simulink model "BLAC_MotorCtrl_Math"  (R2023b)
settings: Solver=FixedStepDiscrete  StartTime=0.0  StopTime=0.1  FixedStep=MC_Sim_BaseStep  RelTol=1e-3  EnableMultiTasking=on
values from neighbouring files (symbols this model uses):
  MC_Hardware_Chip_ADCResultBit = 0.0    [MotorControlDataDictionary_Math.sldd]
  MC_Hardware_Chip_ADCVoltageMax = 1.0    [MotorControlDataDictionary_Math.sldd]
  MC_Hardware_Chip_ADCVoltageRefence = 0.0    [MotorControlDataDictionary_Math.sldd]
  MC_Hardware_Chip_CSAGain = 1.0    [MotorControlDataDictionary_Math.sldd]
  MC_Hardware_Sample_Resistor = 0.001    [MotorControlDataDictionary_Math.sldd]
  MC_MotorModel_Machine_Damp = 0.0    [MotorControlDataDictionary_Math.sldd]
  MC_MotorModel_Machine_Ineria = 0.0    [MotorControlDataDictionary_Math.sldd]
  MC_MotorModel_Machine_Tfric = 0.0    [MotorControlDataDictionary_Math.sldd]
  MC_MotorModel_Rotor_Pn = 4.0    [MotorControlDataDictionary_Math.sldd]
  MC_MotorModel_Stator_Ld = 0.0    [MotorControlDataDictionary_Math.sldd]
  MC_MotorModel_Stator_Lq = 0.0    [MotorControlDataDictionary_Math.sldd]
  MC_MotorModel_Stator_Rs = 1.0    [MotorControlDataDictionary_Math.sldd]
  MC_Sim_BaseStep = 2.5E-8    [MotorControlDataDictionary_Math.sldd]
  MC_Sim_HFTStep = 6.6675E-5    [MotorControlDataDictionary_Math.sldd]
undefined symbols (not defined in the file or in its folder): MC_MOS_DeadTime, MC_Motor_Phi, MC_Motor_Rotor_Pn, MC_Motor_Stator_Ld, MC_Motor_Stator_Lq, MC_Motor_Stator_Rs, MC_Param_CurrentPI_Ki, MC_Param_CurrentPI_Kp, MC_Param_CurrentPI_UdInteMax, MC_Param_CurrentPI_UdInteMin, MC_Param_CurrentPI_UdMax, MC_Param_CurrentPI_UdMin, MC_Param_CurrentPI_UqInteMax, MC_Param_CurrentPI_UqInteMin, MC_Param_CurrentPI_UqMax, MC_Param_CurrentPI_UqMin, MC_Param_Flux_Gamma, MC_Param_Flux_Lalpha, MC_Param_Flux_Lbeta, MC_Param_Flux_Ralpha, MC_Param_Flux_Rbeta, MC_Param_Luen_BEMFalpha, MC_Param_Luen_BEMFbeta, MC_Param_Luen_BEMFErr, MC_Param_Luen_Currentalpha, MC_Param_Luen_Currentbeta, MC_Param_Luen_CurrentErr, MC_Param_Luen_PLL_Ki, MC_Param_Luen_PLL_Kp, MC_Param_Luen_Voltagealpha, MC_Param_Luen_Voltagebeta, MC_Param_PhasetoReal, MC_Param_SMO_CoffA, MC_Param_SMO_CoffB, MC_Param_SpeedtoTheta, MC_Param_SVPWM_DutyMax, MC_Param_SVPWM_DutyMin, MC_Param_SVPWM_SampleOffset1, MC_Param_SVPWM_SampleOffset2, MC_Param_SVPWM_SampleValid
libraries: simulink x29, spsSeriesRLCBranchLib x6, spsVoltageMeasurementLib x6, spsIGBTLib x6, spsDiodeLib x4, spsACVoltageSourceLib x1, spsGroundLib x1, spsPermanentMagnetSynchronousMachineLib x1, spsThreePhaseVIMeasurementLib x1, spspowerguiLib x1
(part 2 of 3)

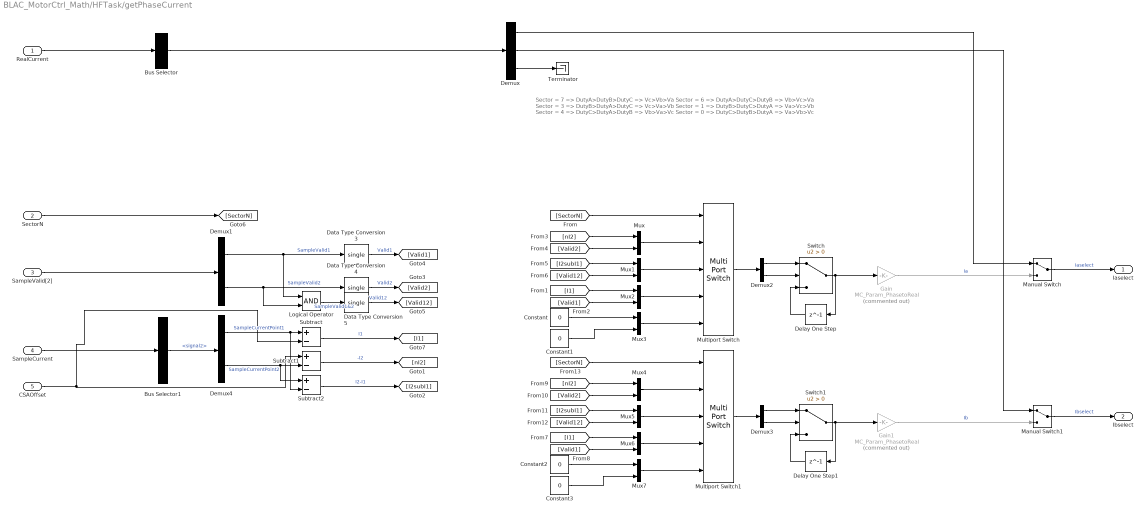
== system BLAC_MotorCtrl_Math/HFTask/getPhaseCurrent ==
  note: Sector = 7 => DutyA>DutyB>DutyC => Vc>Vb>Va
      | Sector = 6 => DutyA>DutyC>DutyB => Vb>Vc>Va
      | Sector = 3 => DutyB>DutyA>DutyC => Vc>Va>Vb
      | Sector = 1 => DutyB>DutyC>DutyA => Va>Vc>Vb
      | Sector = 4 => DutyC>DutyA>DutyB => Vb>Va>Vc
      | Sector = 0 => DutyC>DutyB>DutyA => Va>Vb>Vc
  RealCurrent : Inport
  SectorN : Inport  Port=2
  SampleValid[2] : Inport  Port=3
  SampleCurrent : Inport  Port=4
  CSAOffset : Inport  Port=5
  Bus Selector : BusSelector  OutputSignals=PhaseI  OutputAsBus=on
  Bus Selector1 : BusSelector  OutputSignals=signal2
  Constant{,1..3} (4 alike) : Constant  Value=0  OutDataTypeStr=single
  Data Type Conversion3 : DataTypeConversion  OutDataTypeStr=single  RndMeth=Simplest  SaturateOnIntegerOverflow=off
  Data Type Conversion4 : DataTypeConversion  OutDataTypeStr=single  RndMeth=Simplest  SaturateOnIntegerOverflow=off
  Data Type Conversion5 : DataTypeConversion  OutDataTypeStr=single  RndMeth=Simplest  SaturateOnIntegerOverflow=off
  Delay One Step : Delay  DelayLength=1
  Delay One Step1 : Delay  DelayLength=1
  Demux : Demux  Outputs=3
  Demux{1..4} (4 alike) : Demux  Outputs=2
  Gain : Gain  Commented=on  Gain=MC_Param_PhasetoReal
  Gain1 : Gain  Commented=on  Gain=MC_Param_PhasetoReal
  Logical Operator : Logic  AllPortsSameDT=off  OutDataTypeStr=boolean
  Manual Switch : ManualSwitch
  Manual Switch1 : ManualSwitch
  Multiport Switch : MultiPortSwitch  DataPortOrder=Specify indices  DataPortIndices={[7,6],[3,4],[0,1]}  DataPortForDefault=Additional data port  SaturateOnIntegerOverflow=off  InputSameDT=off
  Multiport Switch1 : MultiPortSwitch  DataPortOrder=Specify indices  DataPortIndices={[3,1],[7,0],[6,4]}  DataPortForDefault=Additional data port  SaturateOnIntegerOverflow=off  InputSameDT=off
  Mux{,1..7} (8 alike) : Mux  Inputs=2
  Subtract : Sum  Inputs=+-
  Subtract1 : Sum  Inputs=+-
  Subtract2 : Sum  Inputs=+-
  Switch : Switch  Criteria=u2 > Threshold  SaturateOnIntegerOverflow=off  InputSameDT=off
  Switch1 : Switch  Criteria=u2 > Threshold  SaturateOnIntegerOverflow=off  InputSameDT=off
  Terminator : Terminator
  Iaselect : Outport
  Ibselect : Outport  Port=2
  wires:
  RealCurrent/1 -> Bus Selector/1
  Bus Selector/1 -> Demux/1
  Manual Switch/1 -> Iaselect/1  "Iaselect"
  Demux/3 -> Terminator/1
  Manual Switch1/1 -> Ibselect/1  "Ibselect"
  Multiport Switch1/1 -> Demux3/1
  Demux3/2 -> Switch1/2
  Demux3/1 -> Switch1/1
  Switch1/1 -> Delay One Step1/1, Gain1/1
  Delay One Step1/1 -> Switch1/3
  Gain1/1 -> Manual Switch1/2  "Ib"
  Gain/1 -> Manual Switch/2  "Ia"
  Delay One Step/1 -> Switch/3
  Switch/1 -> Gain/1, Delay One Step/1
  Demux2/1 -> Switch/1
  Demux2/2 -> Switch/2
  Multiport Switch/1 -> Demux2/1
  [SectorN] -> Multiport Switch1/1
  Mux4/1 -> Multiport Switch1/2
  Mux5/1 -> Multiport Switch1/3
  Mux6/1 -> Multiport Switch1/4
  [I1] -> Mux6/1
  [Valid1] -> Mux6/2
  [nI2] -> Mux4/1
  [Valid2] -> Mux4/2
  [Valid12] -> Mux5/2
  [I2subI1] -> Mux5/1
  Mux7/1 -> Multiport Switch1/5
  Constant2/1 -> Mux7/1
  Constant3/1 -> Mux7/2
  Subtract/1 -> [I1]  "I1"
  Subtract1/1 -> [nI2]  "-I2"
  Data Type Conversion5/1 -> [Valid12]  "Valid12"
  Data Type Conversion4/1 -> [Valid2]  "Valid2"
  Data Type Conversion3/1 -> [Valid1]  "Valid1"
  Subtract2/1 -> [I2subI1]  "I2-I1"
  Constant1/1 -> Mux3/2
  Constant/1 -> Mux3/1
  Mux3/1 -> Multiport Switch/5
  [I2subI1] -> Mux1/1
  [Valid12] -> Mux1/2
  [Valid2] -> Mux/2
  [nI2] -> Mux/1
  [Valid1] -> Mux2/2
  [I1] -> Mux2/1
  [SectorN] -> Multiport Switch/1
  SectorN/1 -> [SectorN]
  Mux2/1 -> Multiport Switch/4
  Mux1/1 -> Multiport Switch/3
  Mux/1 -> Multiport Switch/2
  Logical Operator/1 -> Data Type Conversion5/1  "SampleValid1&2"
  Demux1/2 -> Data Type Conversion4/1, Logical Operator/2  "SampleValid2"
  Demux1/1 -> Data Type Conversion3/1, Logical Operator/1  "SampleValid1"
  SampleValid[2]/1 -> Demux1/1
  Demux4/2 -> Subtract2/1, Subtract1/2  "SampleCurrentPoint2"
  CSAOffset/1 -> Subtract1/1, Subtract/2
  Demux4/1 -> Subtract2/2, Subtract/1  "SampleCurrentPoint1"
  Bus Selector1/1 -> Demux4/1  "<signal2>"
  SampleCurrent/1 -> Bus Selector1/1
  Demux/1 -> Manual Switch/1
  Demux/2 -> Manual Switch1/1

== system BLAC_MotorCtrl_Math/HFTask/getSinCos ==
  Theta : Inport
  Sin : Trigonometry
  Sin1 : Trigonometry  Operator=cos
  SinTheta : Outport
  CosTheta : Outport  Port=2
  wires:
  Theta/1 -> Sin1/1, Sin/1
  Sin/1 -> SinTheta/1
  Sin1/1 -> CosTheta/1

== system BLAC_MotorCtrl_Math/HFTask/invParkTransform ==
  Ud : Inport
  Uq : Inport  Port=2
  SinTheta : Inport  Port=3
  CosTheta : Inport  Port=4
  Add : Sum
  Product{,1..3} (4 alike) : Product
  Subtract : Sum  Inputs=+-
  Ualpha : Outport
  Ubeta : Outport  Port=2
  wires:
  Uq/1 -> Product3/1, Product1/1
  Subtract/1 -> Ualpha/1  "Ualpha"
  CosTheta/1 -> Product/2, Product3/2
  SinTheta/1 -> Product2/2, Product1/2
  Product/1 -> Subtract/1
  Product1/1 -> Subtract/2
  Ud/1 -> Product/1, Product2/1
  Product2/1 -> Add/1
  Product3/1 -> Add/2
  Add/1 -> Ubeta/1  "Ubeta"

== system BLAC_MotorCtrl_Math/HFTask/karmalObservor ==
  In1 : Inport
  Out1 : Outport
  wires:
  In1/1 -> Out1/1

== system BLAC_MotorCtrl_Math/HFTask/scvmobservor ==
  Vd : Inport
  Vq : Inport  Port=2
  Id : Inport  Port=3
  Iq : Inport  Port=4
  getW : Subsystem
  wires:
  Vd/1 -> getW/1(Vd)
  Vq/1 -> getW/2(Vq)
  Id/1 -> getW/3(Id)
  Iq/1 -> getW/4(Iq)

== system BLAC_MotorCtrl_Math/HFTask/smo ==
  Valpha : Inport
  Vbeta : Inport  Port=2
  Ialpha : Inport  Port=3
  Ibeta : Inport  Port=4
  getE : Subsystem
  getSpeedandTheta : Subsystem
  Speed : Outport
  Theta : Outport  Port=2
  wires:
  Valpha/1 -> getE/1(Valpha)
  Vbeta/1 -> getE/2(Vbeta)
  Ialpha/1 -> getE/3(Ialpha)
  Ibeta/1 -> getE/4(Ibeta)
  getE/1(Ealpha) -> getSpeedandTheta/1(Ealpha)
  getE/2(Ebeta) -> getSpeedandTheta/2(Ebeta)
  getSpeedandTheta/1(Speed) -> Speed/1
  getSpeedandTheta/2(Theta) -> Theta/1

== system BLAC_MotorCtrl_Math/HFTask/svpwm ==
  Valpha : Inport
  Vbeta : Inport  Port=2
  Vdc : Inport  Port=3
  Ia : Inport  Port=4
  Ib : Inport  Port=5
  PhaseShortEnableFlag : Inport  Port=6
  Terminator : Terminator
  getVoltageExchange : Subsystem
  setDTCompelte : Subsystem
  setPhaseandSample_ORS_Double : Subsystem
  setPhaseandSample_ORS_Double1 : Subsystem  Commented=on
  DutySVPWM : Outport
  SamplePoint : Outport  Port=2
  SampleValid : Outport  Port=3
  SectorN : Outport  Port=4
  wires:
  Valpha/1 -> getVoltageExchange/1(Valpha)
  Vbeta/1 -> getVoltageExchange/2(Vbeta)
  Vdc/1 -> getVoltageExchange/3(Vdc)
  getVoltageExchange/1(Va) -> setDTCompelte/1(Va)
  getVoltageExchange/2(Vb) -> setDTCompelte/2(Vb)
  getVoltageExchange/3(Vc) -> setDTCompelte/3(Vc)
  getVoltageExchange/4(Vmed) -> setDTCompelte/4(Vmed)
  Ia/1 -> setDTCompelte/5(Ia)
  Ib/1 -> setDTCompelte/6(ib)
  setDTCompelte/1(SectorN) -> SectorN/1, setPhaseandSample_ORS_Double/1(SectorN)
  setDTCompelte/2(DutyLMS) -> setPhaseandSample_ORS_Double/2(DutyLMS)
  setPhaseandSample_ORS_Double/1(DutySVPWM) -> DutySVPWM/1
  setPhaseandSample_ORS_Double/2(SamplePoint) -> SamplePoint/1
  setPhaseandSample_ORS_Double/3(SampleValid) -> SampleValid/1
  PhaseShortEnableFlag/1 -> Terminator/1

== system BLAC_MotorCtrl_Math/HFTask/voltageLimit ==
  UdRef : Inport
  UqRef : Inport  Port=2
  Umax : Inport  Port=3
  Add : Sum
  Compare To Constant : simulink/Logic and Bit Operations/Compare To Constant  relop=<=  const=0  OutDataTypeStr=boolean
  Compare To Constant1 : simulink/Logic and Bit Operations/Compare To Constant  relop=>=  const=0  OutDataTypeStr=boolean
  Constant : Constant  Value=0  OutDataTypeStr=single
  Gain : Gain  Gain=-1
  Gain1 : Gain  Gain=-1
  Product : Product
  Saturation Dynamic : simulink/Discontinuities/Saturation Dynamic  OutMin=[]  OutMax=[]  OutDataTypeStr=Inherit: Same as second input  OutDataType=fixdt(1, 16)  OutScaling=2^-10  DoSatur=off
  Sqrt : Sqrt
  Subtract : Sum  Inputs=+-
  Switch : Switch  Criteria=u2 > Threshold  SaturateOnIntegerOverflow=off  InputSameDT=off
  Switch1 : Switch  Criteria=u2 > Threshold  SaturateOnIntegerOverflow=off  InputSameDT=off
  Switch2 : Switch  Criteria=u2 > Threshold  SaturateOnIntegerOverflow=off  InputSameDT=off
  Ud : Outport
  Uq : Outport  Port=2
  wires:
  Add/1 -> Product/1
  Subtract/1 -> Product/2
  Product/1 -> Compare To Constant/1, Sqrt/1
  Compare To Constant/1 -> [UdOverFlow]
  Sqrt/1 -> Gain/1, Saturation Dynamic/1
  Gain/1 -> Saturation Dynamic/3
  UdRef/1 -> [UdRef]
  UqRef/1 -> [UqRef]
  Umax/1 -> [Umax]
  [Umax] -> Subtract/1, Add/1
  [UdRef] -> Add/2, Subtract/2
  [UqRef] -> Saturation Dynamic/2
  Saturation Dynamic/1 -> Switch/3
  [UdOverFlow] -> Switch/2
  Constant/1 -> Switch/1
  Switch/1 -> Uq/1  "UqLimit"
  Switch1/1 -> Ud/1  "UdLimit"
  Switch2/1 -> Switch1/1
  [UdRef] -> Compare To Constant1/1
  Compare To Constant1/1 -> Switch2/2
  [Umax] -> Gain1/1, Switch2/1
  Gain1/1 -> Switch2/3
  [UdOverFlow] -> Switch1/2
  [UdRef] -> Switch1/3

== system BLAC_MotorCtrl_Math/Hardware_Sim/ACtoDC_Sim ==
  Diode{1..4} (4 alike) : spsDiodeLib/Diode  Ron=MC_Hardware_Diode_Rds  Lon=MC_Hardware_Diode_Lon  Vf=MC_Hardware_Diode_Vf  IC=0  UseSnubber=0  Rs=MC_Hardware_Diode_SR  Cs=MC_Hardware_Diode_SC  Measurements=off
  U : PMIOPort  Side=Left
  L : PMIOPort  Port=2  Side=Left
  VH : PMIOPort  Port=3  Side=Right
  VL : PMIOPort  Port=4  Side=Right
  connections:
  L/RConn1 -- Diode3/RConn1 -- Diode2/LConn1
  VL/RConn1 -- Diode4/LConn1 -- Diode3/LConn1
  Diode1/RConn1 -- Diode2/RConn1 -- VH/RConn1
  Diode1/LConn1 -- Diode4/RConn1 -- U/RConn1

== system BLAC_MotorCtrl_Math/Hardware_Sim/CurrentSample_Sim ==
  Current_Sample_Trigger : Inport
  ADCSample_Sim : Subsystem  Commented=on
  PhaseCurrentSmaple : Subsystem  Variant=on  VariantControl=PhaseCurrentSmaple
  Series RLC Branch{,1..3} (4 alike) : spsSeriesRLCBranchLib/Series RLC Branch  LConnTagsString=__new0  RConnTagsString=__new0  BranchType=R  Resistance=MC_Hardware_Sample_Resistor  Inductance=1e-3  SetiL0=off  InitialCurrent=0  Capacitance=1e-6  Setx0=off  InitialVoltage=0  Measurements=None
  Voltage Measurement{,1..3} (4 alike) : spsVoltageMeasurementLib/Voltage Measurement  PhasorSimulation=off  OutputType=Complex  PSBequivalent=0
  AL : PMIOPort  Side=Left
  BL : PMIOPort  Port=2  Side=Left
  CL : PMIOPort  Port=3  Side=Left
  VL : PMIOPort  Port=4  Side=Left
  Current_Sample : Outport
  wires:
  Voltage Measurement1/1 -> PhaseCurrentSmaple/4(SRV_A)
  Voltage Measurement2/1 -> PhaseCurrentSmaple/3(SRV_B)
  Voltage Measurement3/1 -> PhaseCurrentSmaple/2(SRV_C)
  Voltage Measurement/1 -> PhaseCurrentSmaple/5(ShuntV)
  Current_Sample_Trigger/1 -> PhaseCurrentSmaple/1(SampleTrigger)
  PhaseCurrentSmaple/1(CurrentSampleResult) -> Current_Sample/1
  connections:
  Series RLC Branch1/RConn1 -- Voltage Measurement1/LConn2 -- Voltage Measurement3/LConn2 -- Series RLC Branch3/RConn1 -- Voltage Measurement2/LConn2 -- Series RLC Branch2/RConn1 -- Voltage Measurement/LConn1 -- Series RLC Branch/LConn1
  Series RLC Branch2/LConn1 -- Voltage Measurement2/LConn1 -- BL/RConn1
  Series RLC Branch1/LConn1 -- Voltage Measurement1/LConn1 -- AL/RConn1
  VL/RConn1 -- Voltage Measurement/LConn2 -- Series RLC Branch/RConn1
  Series RLC Branch3/LConn1 -- Voltage Measurement3/LConn1 -- CL/RConn1

== system BLAC_MotorCtrl_Math/Hardware_Sim/DrivePWM_Sim ==
  ClockCounter : Inport
  DrivePWM : Inport  Port=2
  Data Type Conversion{,1..5} (6 alike) : DataTypeConversion  OutDataTypeStr=double  RndMeth=Simplest  SaturateOnIntegerOverflow=off
  Demux : Demux  Outputs=6
  Relational Operator : RelationalOperator  Operator=>  OutDataTypeStr=boolean  RndMeth=Simplest  InputSameDT=off
  Relational Operator1 : RelationalOperator  Operator=>  OutDataTypeStr=boolean  RndMeth=Simplest  InputSameDT=off
  Relational Operator2 : RelationalOperator  Operator=>  OutDataTypeStr=boolean  RndMeth=Simplest  InputSameDT=off
  Relational Operator3 : RelationalOperator  Operator=<  OutDataTypeStr=boolean  RndMeth=Simplest  InputSameDT=off
  Relational Operator4 : RelationalOperator  Operator=<  OutDataTypeStr=boolean  RndMeth=Simplest  InputSameDT=off
  Relational Operator5 : RelationalOperator  Operator=<  OutDataTypeStr=boolean  RndMeth=Simplest  InputSameDT=off
  Drive_A_H : Outport
  Drive_B_H : Outport  Port=2
  Drive_C_H : Outport  Port=3
  Drive_A_L : Outport  Port=4
  Drive_B_L : Outport  Port=5
  Drive_C_L : Outport  Port=6
  wires:
  Relational Operator1/1 -> Data Type Conversion1/1
  Demux/2 -> Relational Operator1/2
  Demux/5 -> Relational Operator4/2
  Demux/1 -> Relational Operator/2
  DrivePWM/1 -> Demux/1
  Relational Operator2/1 -> Data Type Conversion3/1
  ClockCounter/1 -> Relational Operator5/1, Relational Operator4/1, Relational Operator3/1, Relational Operator2/1, Relational Operator1/1, Relational Operator/1
  Demux/6 -> Relational Operator5/2
  Relational Operator/1 -> Data Type Conversion/1
  Demux/4 -> Relational Operator3/2
  Relational Operator3/1 -> Data Type Conversion2/1
  Data Type Conversion5/1 -> Drive_C_L/1
  Relational Operator5/1 -> Data Type Conversion5/1
  Demux/3 -> Relational Operator2/2
  Relational Operator4/1 -> Data Type Conversion4/1
  Data Type Conversion3/1 -> Drive_C_H/1
  Data Type Conversion4/1 -> Drive_B_L/1
  Data Type Conversion2/1 -> Drive_A_L/1
  Data Type Conversion1/1 -> Drive_B_H/1
  Data Type Conversion/1 -> Drive_A_H/1

== system BLAC_MotorCtrl_Math/Hardware_Sim/IGBT_Drive_Sim ==
  Drive_A_H : Inport
  Drive_B_H : Inport  Port=2
  Drive_C_H : Inport  Port=3
  Drive_A_L : Inport  Port=4
  Drive_B_L : Inport  Port=5
  Drive_C_L : Inport  Port=6
  IGBT{,1..5} (6 alike) : spsIGBTLib/IGBT  Ron=MC_Hardware_IGBT_Rds  Lon=MC_Hardware_IGBT_Lon  Vf=MC_Hardware_IGBT_Vf  Tf=1e-6  Tt=2e-6  IC=0  Rs=MC_Hardware_IGBT_SR  Cs=MC_Hardware_IGBT_SC  Measurements=on
  Mux : Mux  Inputs=3
  Mux1 : Mux  Inputs=3
  VH : PMIOPort  Side=Left
  A : PMIOPort  Port=2  Side=Right
  B : PMIOPort  Port=3  Side=Right
  C : PMIOPort  Port=4  Side=Right
  AL : PMIOPort  Port=5  Side=Right
  BL : PMIOPort  Port=6  Side=Right
  CL : PMIOPort  Port=7  Side=Right
  IGBT_M_H : Outport
  IGBT_M_L : Outport  Port=2
  wires:
  IGBT4/1 -> Mux/2
  Drive_C_H/1 -> IGBT2/1
  Drive_B_H/1 -> IGBT1/1
  IGBT5/1 -> Mux/1
  Drive_B_L/1 -> IGBT4/1
  Drive_A_H/1 -> IGBT/1
  Drive_C_L/1 -> IGBT5/1
  IGBT3/1 -> Mux/3
  Drive_A_L/1 -> IGBT3/1
  IGBT2/1 -> Mux1/3
  IGBT1/1 -> Mux1/2
  IGBT/1 -> Mux1/1
  Mux1/1 -> IGBT_M_H/1
  Mux/1 -> IGBT_M_L/1
  connections:
  IGBT/RConn1 -- IGBT3/LConn1 -- A/RConn1
  IGBT3/RConn1 -- AL/RConn1
  IGBT2/LConn1 -- IGBT1/LConn1 -- VH/RConn1 -- IGBT/LConn1
  C/RConn1 -- IGBT5/LConn1 -- IGBT2/RConn1
  B/RConn1 -- IGBT4/LConn1 -- IGBT1/RConn1
  IGBT5/RConn1 -- CL/RConn1
  IGBT4/RConn1 -- BL/RConn1

== system BLAC_MotorCtrl_Math/Hardware_Sim/SampleTrigger_Sim ==
  ClockCounter : Inport
  SamplePoint : Inport  Port=2
  Data Type Conversion{,1..4} (5 alike) : DataTypeConversion  OutDataTypeStr=double  RndMeth=Simplest  SaturateOnIntegerOverflow=off
  Demux : Demux  Outputs=5
  Mux : Mux  Inputs=3
  Relational Operator{,1..4} (5 alike) : RelationalOperator  Operator=>  OutDataTypeStr=boolean  RndMeth=Simplest  InputSameDT=off
  Current_Sample_Trigger : Outport
  Vbus_Sample_Trigger : Outport  Port=2
  Temp_Sample_Trigger : Outport  Port=3
  wires:
  SamplePoint/1 -> Demux/1
  Relational Operator/1 -> Data Type Conversion/1
  Demux/1 -> Relational Operator/2
  Demux/2 -> Relational Operator1/2
  Relational Operator1/1 -> Data Type Conversion1/1
  Relational Operator2/1 -> Data Type Conversion2/1
  Demux/4 -> Relational Operator2/2
  Demux/5 -> Relational Operator3/2
  Relational Operator3/1 -> Data Type Conversion3/1
  ClockCounter/1 -> Relational Operator4/1, Relational Operator3/1, Relational Operator2/1, Relational Operator1/1, Relational Operator/1
  Data Type Conversion/1 -> Mux/1
  Data Type Conversion1/1 -> Mux/2
  Mux/1 -> Current_Sample_Trigger/1
  Data Type Conversion2/1 -> Vbus_Sample_Trigger/1
  Data Type Conversion3/1 -> Temp_Sample_Trigger/1
  Demux/3 -> Relational Operator4/2
  Relational Operator4/1 -> Data Type Conversion4/1
  Data Type Conversion4/1 -> Mux/3

== system BLAC_MotorCtrl_Math/Hardware_Sim/VbusSample_Sim ==
  Vbus_Sample_Trigger : Inport
  ADCSample_Sim : Subsystem
  ADCSample_Sim1 : Subsystem
  Add1 : Sum
  Add2 : Sum
  Band-Limited White Noise : simulink/Sources/Band-Limited White Noise  Cov=MC_Sim_NoisePower_VACbus  Ts=MC_Sim_BaseStep  seed=[23222]
  Band-Limited White Noise1 : simulink/Sources/Band-Limited White Noise  Cov=MC_Sim_NoisePower_VDCbus  Ts=MC_Sim_BaseStep  seed=[23241]
  Series RLC Branch : spsSeriesRLCBranchLib/Series RLC Branch  LConnTagsString=__new0  RConnTagsString=__new0  BranchType=R  Resistance=1e3  Inductance=1e-3  SetiL0=off  InitialCurrent=0  Capacitance=1e-6  Setx0=off  InitialVoltage=0  Measurements=None
  Series RLC Branch1 : spsSeriesRLCBranchLib/Series RLC Branch  LConnTagsString=__new0  RConnTagsString=__new0  BranchType=R  Resistance=1e3  Inductance=1e-3  SetiL0=off  InitialCurrent=0  Capacitance=1e-6  Setx0=off  InitialVoltage=0  Measurements=None
  Voltage Measurement : spsVoltageMeasurementLib/Voltage Measurement  PhasorSimulation=off  OutputType=Complex  PSBequivalent=0
  Voltage Measurement1 : spsVoltageMeasurementLib/Voltage Measurement  PhasorSimulation=off  OutputType=Complex  PSBequivalent=0
  DCH : PMIOPort  Side=Left
  DCL : PMIOPort  Port=2  Side=Left
  ACH : PMIOPort  Port=3  Side=Left
  ACL : PMIOPort  Port=4  Side=Left
  Vbus_Sample_AC : Outport
  Vbus_Sample_DC : Outport  Port=2
  wires:
  ADCSample_Sim/1(Sample_Out) -> Vbus_Sample_AC/1
  ADCSample_Sim1/1(Sample_Out) -> Vbus_Sample_DC/1
  Vbus_Sample_Trigger/1 -> ADCSample_Sim1/Trigger, ADCSample_Sim/Trigger
  Band-Limited White Noise/1 -> Add1/2
  Add1/1 -> ADCSample_Sim/1(Sample_In)
  Voltage Measurement/1 -> Add1/1
  Band-Limited White Noise1/1 -> Add2/2
  Voltage Measurement1/1 -> Add2/1
  Add2/1 -> ADCSample_Sim1/1(Sample_In)
  connections:
  ACH/RConn1 -- Voltage Measurement/LConn1 -- Series RLC Branch/LConn1
  ACL/RConn1 -- Voltage Measurement/LConn2 -- Series RLC Branch/RConn1
  DCL/RConn1 -- Series RLC Branch1/RConn1 -- Voltage Measurement1/LConn2
  DCH/RConn1 -- Series RLC Branch1/LConn1 -- Voltage Measurement1/LConn1

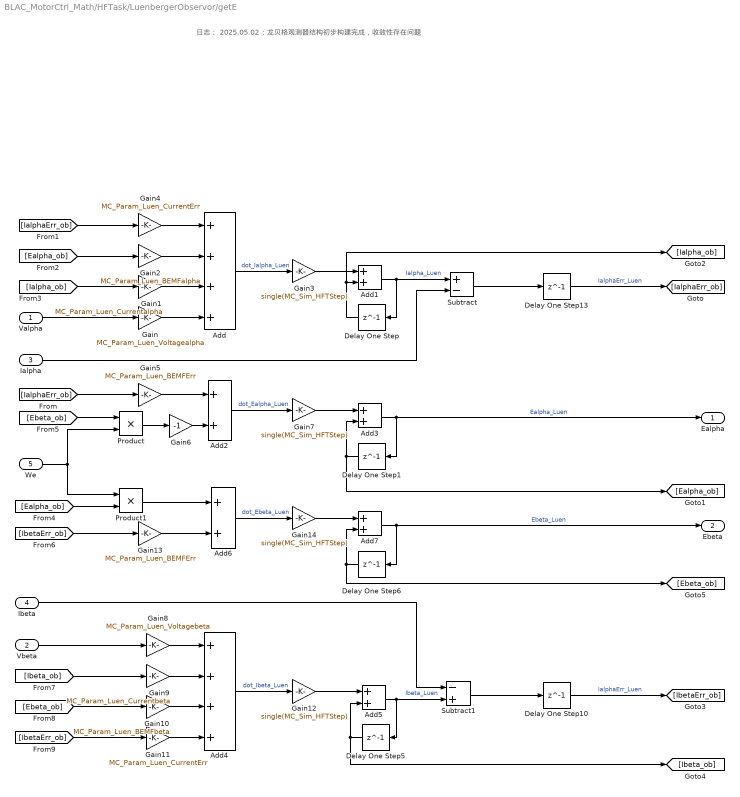
== system BLAC_MotorCtrl_Math/HFTask/LuenbergerObservor/getE ==
  note: 日志：
      | 2025.05.02：龙贝格观测器结构初步构建完成，收敛性存在问题
  Valpha : Inport
  Vbeta : Inport  Port=2
  Ialpha : Inport  Port=3
  Ibeta : Inport  Port=4
  We : Inport  Port=5
  Add : Sum  Inputs=++++
  Add{1..3,5..7} (6 alike) : Sum
  Add4 : Sum  Inputs=++++
  Delay One Step{,1,5..6,10,13} (6 alike) : Delay  DelayLength=1
  Gain : Gain  Gain=MC_Param_Luen_Voltagealpha
  Gain1 : Gain  Gain=MC_Param_Luen_Currentalpha
  Gain10 : Gain  Gain=MC_Param_Luen_BEMFbeta
  Gain11 : Gain  Gain=MC_Param_Luen_CurrentErr
  Gain{3,7,12,14} (4 alike) : Gain  Gain=single(MC_Sim_HFTStep)
  Gain13 : Gain  Gain=MC_Param_Luen_BEMFErr
  Gain2 : Gain  Gain=MC_Param_Luen_BEMFalpha
  Gain4 : Gain  Gain=MC_Param_Luen_CurrentErr
  Gain5 : Gain  Gain=MC_Param_Luen_BEMFErr
  Gain6 : Gain  Gain=-1
  Gain8 : Gain  Gain=MC_Param_Luen_Voltagebeta
  Gain9 : Gain  Gain=MC_Param_Luen_Currentbeta
  Product : Product
  Product1 : Product
  Subtract : Sum  Inputs=+-
  Subtract1 : Sum  Inputs=-+
  Ealpha : Outport
  Ebeta : Outport  Port=2
  wires:
  Valpha/1 -> Gain/1
  Add/1 -> Gain3/1  "dot_Ialpha_Luen"
  Gain2/1 -> Add/2
  Gain1/1 -> Add/3
  Gain/1 -> Add/4
  Gain4/1 -> Add/1
  Gain3/1 -> Add1/1
  Add1/1 -> Subtract/1, Delay One Step/1  "Ialpha_Luen"
  Delay One Step/1 -> [Ialpha_ob], Add1/2
  Ialpha/1 -> Subtract/2
  Subtract/1 -> Delay One Step13/1
  [IalphaErr_ob] -> Gain5/1
  Gain5/1 -> Add2/1
  Gain6/1 -> Add2/2
  Add2/1 -> Gain7/1  "dot_Ealpha_Luen"
  Delay One Step1/1 -> Add3/2, [Ealpha_ob]
  Add3/1 -> Ealpha/1, Delay One Step1/1  "Ealpha_Luen"
  Gain7/1 -> Add3/1
  Product/1 -> Gain6/1
  We/1 -> Product/2, Product1/1
  Vbeta/1 -> Gain8/1
  Gain8/1 -> Add4/1
  Gain9/1 -> Add4/2
  Gain10/1 -> Add4/3
  Gain11/1 -> Add4/4
  [IalphaErr_ob] -> Gain4/1
  [Ealpha_ob] -> Gain2/1
  [Ialpha_ob] -> Gain1/1
  Add4/1 -> Gain12/1  "dot_Ibeta_Luen"
  Delay One Step5/1 -> Add5/2, [Ibeta_ob]
  Add5/1 -> Subtract1/2, Delay One Step5/1  "Ibeta_Luen"
  Gain12/1 -> Add5/1
  Ibeta/1 -> Subtract1/1
  Subtract1/1 -> Delay One Step10/1
  Add6/1 -> Gain14/1  "dot_Ebeta_Luen"
  Gain13/1 -> Add6/2
  Product1/1 -> Add6/1
  Gain14/1 -> Add7/1
  Add7/1 -> Ebeta/1, Delay One Step6/1  "Ebeta_Luen"
  Delay One Step6/1 -> Add7/2, [Ebeta_ob]
  [Ealpha_ob] -> Product1/2
  [Ebeta_ob] -> Product/1
  [IbetaErr_ob] -> Gain13/1
  [Ibeta_ob] -> Gain9/1
  [IbetaErr_ob] -> Gain11/1
  [Ebeta_ob] -> Gain10/1
  Delay One Step13/1 -> [IalphaErr_ob]  "IalphaErr_Luen"
  Delay One Step10/1 -> [IbetaErr_ob]  "IalphaErr_Luen"

== system BLAC_MotorCtrl_Math/HFTask/LuenbergerObservor/getSpeedandTheta ==
  note: 日志：
      | 2025.03.19：反电势正负号识别错误，改正后可以使用
  Ealpha : Inport
  Ebeta : Inport  Port=2
  Add : Sum
  Add1 : Sum
  Add2 : Sum
  Constant : Constant  Value=2*pi  OutDataTypeStr=single
  Delay One Step : Delay  DelayLength=1
  Delay One Step2 : Delay  DelayLength=1
  Gain1 : Gain  Gain=MC_Param_Luen_PLL_Kp
  Gain2 : Gain  Gain=MC_Param_Luen_PLL_Ki
  Gain3 : Gain  Gain=MC_Param_SpeedtoTheta
  Gain5 : Gain  Gain=30/(pi*MC_Motor_Rotor_Pn)  OutDataTypeStr=single  RndMeth=Simplest
  Mod : Math  Operator=mod
  Product : Product
  Product1 : Product
  Sin : Trigonometry  OutputSignalType=real
  Sin1 : Trigonometry  Operator=cos  OutputSignalType=real
  Subtract : Sum  Inputs=+-
  Speed : Outport
  Theta : Outport  Port=2
  We : Outport  Port=3
  wires:
  Gain5/1 -> Speed/1  "SpeedLuen_RPM"
  Product1/1 -> Subtract/2  "LuenCos"
  Product/1 -> Subtract/1  "LuenSin"
  [Theta_Last] -> Sin/1, Sin1/1
  Add1/1 -> We/1, Gain3/1, Gain5/1  "WeLuen"
  Mod/1 -> Delay One Step2/1, Theta/1  "ThetaLuen"
  Delay One Step2/1 -> [Theta_Last], Add2/2
  Constant/1 -> Mod/2
  Add2/1 -> Mod/1
  Gain3/1 -> Add2/1
  Subtract/1 -> Gain1/1, Gain2/1  "LuenErr"
  Gain1/1 -> Add1/1
  Delay One Step/1 -> Add/2
  Add/1 -> Add1/2, Delay One Step/1
  Gain2/1 -> Add/1
  Sin/1 -> Product1/2
  Sin1/1 -> Product/2
  Ealpha/1 -> Product1/1
  Ebeta/1 -> Product/1

== system BLAC_MotorCtrl_Math/HFTask/currentADRC/LESO ==
  Id : Inport
  Ud : Inport  Port=2
  Iq : Inport  Port=3
  Uq : Inport  Port=4
  Add1 : Sum  Inputs=+++  AccumDataTypeStr=single  RndMeth=Simplest
  Add{2,4..6} (4 alike) : Sum
  Add3 : Sum  Inputs=+++  AccumDataTypeStr=single  RndMeth=Simplest
  Delay{,1..3} (4 alike) : Delay  DelayLength=1  InitialCondition=single(0)
  Gain1 : Gain  Gain=2*pi*100*2*pi*100
  Gain2 : Gain  Gain=2*2*pi*100
  Gain4 : Gain  Gain=2*pi*100*2*pi*100
  Gain5 : Gain  Gain=2*2*pi*100
  Gain6 : Gain  Gain=1/single(MC_Motor_Stator_Ld)
  Gain7 : Gain  Gain=1/single(MC_Motor_Stator_Lq)
  Subtract1 : Sum  Inputs=+-
  Subtract2 : Sum  Inputs=+-
  Ts{1..4} (4 alike) : Gain  Gain=single(MC_Sim_HFTStep)  ParamDataTypeStr=single  OutDataTypeStr=single  RndMeth=Simplest
  falFunc : Subsystem  Commented=on
  Id_ESO : Outport
  Iq_ESO : Outport  Port=2
  Id_Dis : Outport  Port=3
  Iq_Dis : Outport  Port=4
  wires:
  [Id_ESO_Delay] -> Subtract1/2
  Id/1 -> Subtract1/1
  Gain2/1 -> Add3/2
  Ud/1 -> Gain6/1
  Add3/1 -> Ts1/1
  Ts1/1 -> Add4/1
  Add4/1 -> Delay/1, Id_ESO/1  "Id_ESO"
  Delay/1 -> Add4/2, [Id_ESO_Delay]
  Subtract1/1 -> Gain1/1, Gain2/1
  Add5/1 -> Id_Dis/1, Delay1/1  "Id_Dis"
  Gain1/1 -> Ts2/1
  Ts2/1 -> Add5/1
  Delay1/1 -> Add3/3, Add5/2
  Delay3/1 -> Add1/3, Add6/2
  Ts4/1 -> Add6/1
  Gain4/1 -> Ts4/1
  Add6/1 -> Iq_Dis/1, Delay3/1  "Iq_Dis"
  Subtract2/1 -> Gain4/1, Gain5/1
  Delay2/1 -> [Iq_ESO_Delay], Add2/2
  Add2/1 -> Iq_ESO/1, Delay2/1  "Iq_ESO"
  Ts3/1 -> Add2/1
  Add1/1 -> Ts3/1
  Uq/1 -> Gain7/1
  Gain5/1 -> Add1/2
  Iq/1 -> Subtract2/1
  [Iq_ESO_Delay] -> Subtract2/2
  Gain6/1 -> Add3/1  "bUd"
  Gain7/1 -> Add1/1  "bUq"

== system BLAC_MotorCtrl_Math/HFTask/currentADRC/NLSEF ==
  Id_Ref : Inport
  Iq_Ref : Inport  Port=2
  Id_ESO : Inport  Port=3
  Iq_ESO : Inport  Port=4
  Id_ESO_Dis : Inport  Port=5
  Iq_ESO_Dis : Inport  Port=6
  Gain1 : Gain  Gain=0.1  OutDataTypeStr=single  RndMeth=Simplest
  Gain2 : Gain  Gain=0.1  OutDataTypeStr=single  RndMeth=Simplest
  Gain3 : Gain  Gain=single(MC_Motor_Stator_Ld)  OutDataTypeStr=single  RndMeth=Simplest
  Gain5 : Gain  Gain=single(MC_Motor_Stator_Lq)  OutDataTypeStr=single  RndMeth=Simplest
  Saturation : Saturate  UpperLimit=MC_Param_CurrentPI_UdMax  LowerLimit=MC_Param_CurrentPI_UdMin
  Saturation1 : Saturate  UpperLimit=MC_Param_CurrentPI_UqMax  LowerLimit=MC_Param_CurrentPI_UqMin
  Subtract : Sum  Inputs=+-
  Subtract1 : Sum  Inputs=+-  OutDataTypeStr=single  AccumDataTypeStr=single  RndMeth=Simplest
  Subtract2 : Sum  Inputs=+-
  Subtract3 : Sum  Inputs=+-
  Ud_ADRC : Outport
  Uq_ADRC : Outport  Port=2
  wires:
  Id_Ref/1 -> Subtract/1
  Id_ESO/1 -> Subtract/2
  Subtract2/1 -> Saturation/1  "Ud_ADRC"
  Saturation/1 -> Ud_ADRC/1
  Saturation1/1 -> Uq_ADRC/1
  Subtract3/1 -> Saturation1/1  "Uq_ADRC"
  Iq_ESO/1 -> Subtract1/2
  Iq_Ref/1 -> Subtract1/1
  Id_ESO_Dis/1 -> Gain3/1
  Gain3/1 -> Subtract2/2
  Iq_ESO_Dis/1 -> Gain5/1
  Gain5/1 -> Subtract3/2
  Gain2/1 -> Subtract3/1
  Subtract/1 -> Gain1/1  "Id_Err"
  Gain1/1 -> Subtract2/1
  Subtract1/1 -> Gain2/1  "Iq_Err"

== system BLAC_MotorCtrl_Math/HFTask/currentPIRControl/currentRController_D ==
  CurrErr : Inport
  Wm : Inport  Port=2
  UReal : Inport  Port=3
  Add : Sum  Inputs=+---
  Delay One Step : Delay  DelayLength=1  InitialCondition=single(0)
  Delay One Step1 : Delay  InitialCondition=single(0)
  Delay One Step2 : Delay  InitialCondition=single(0)
  Gain{,1..3} (4 alike) : Gain
  Saturation : Saturate
  Terminator : Terminator
  Terminator1 : Terminator
  UR_Ref : Outport
  wires:
  Gain/1 -> Add/1
  CurrErr/1 -> Delay One Step2/1, Gain/1
  Delay One Step2/1 -> Gain1/1
  Gain1/1 -> Add/2
  Wm/1 -> Terminator/1
  UReal/1 -> Terminator1/1
  Add/1 -> Saturation/1
  Delay One Step/1 -> Gain2/1
  Delay One Step1/1 -> Gain3/1
  Gain3/1 -> Add/4
  Gain2/1 -> Add/3
  Saturation/1 -> Delay One Step/1, Delay One Step1/1, UR_Ref/1

== system BLAC_MotorCtrl_Math/HFTask/currentPIRControl/currentRController_Q ==
  CurrErr : Inport
  Wm : Inport  Port=2
  UReal : Inport  Port=3
  Add : Sum  Inputs=+---
  Delay One Step : Delay  DelayLength=1  InitialCondition=single(0)
  Delay One Step1 : Delay  InitialCondition=single(0)
  Delay One Step2 : Delay  InitialCondition=single(0)
  Gain{,1..3} (4 alike) : Gain
  Saturation : Saturate
  Terminator : Terminator
  Terminator1 : Terminator
  UR_Ref : Outport
  wires:
  Saturation/1 -> UR_Ref/1, Delay One Step1/1, Delay One Step/1
  Gain2/1 -> Add/3
  Gain3/1 -> Add/4
  Delay One Step1/1 -> Gain3/1
  Delay One Step/1 -> Gain2/1
  Add/1 -> Saturation/1
  UReal/1 -> Terminator1/1
  Wm/1 -> Terminator/1
  Gain1/1 -> Add/2
  Delay One Step2/1 -> Gain1/1
  CurrErr/1 -> Gain/1, Delay One Step2/1
  Gain/1 -> Add/1

== system BLAC_MotorCtrl_Math/HFTask/fluxobservor/getFlux ==
  note: 日志：
      | 2025.02.28：滑膜观测器建模无问题，但是反电势观测存在问题，暂时分析为参数问题
  Valpha : Inport
  Vbeta : Inport  Port=2
  Ialpha : Inport  Port=3
  Ibeta : Inport  Port=4
  Add{,1..4} (5 alike) : Sum
  Constant : Constant  Value=MC_Motor_Phi  OutDataTypeStr=single
  Delay One Step{,1..3} (4 alike) : Delay  DelayLength=1
  Gain : Gain  Gain=MC_Param_Flux_Ralpha
  Gain1 : Gain  Gain=MC_Param_Flux_Gamma  OutDataTypeStr=single  RndMeth=Simplest
  Gain2 : Gain  Gain=single(MC_Sim_HFTStep)  OutDataTypeStr=single  RndMeth=Simplest
  Gain3 : Gain  Gain=MC_Param_Flux_Lalpha  OutDataTypeStr=single  RndMeth=Simplest
  Gain4 : Gain  Gain=MC_Param_Flux_Rbeta
  Gain5 : Gain  Gain=MC_Param_Flux_Gamma  OutDataTypeStr=single  RndMeth=Simplest
  Gain6 : Gain  Gain=single(MC_Sim_HFTStep)
  Gain7 : Gain  Gain=MC_Param_Flux_Lbeta  OutDataTypeStr=single  RndMeth=Simplest
  Product : Product
  Product1 : Product
  Square : Math  Operator=square
  Square1 : Math  Operator=square
  Square2 : Math  Operator=square
  Subtract{,1..4} (5 alike) : Sum  Inputs=+-
  Phialpha : Outport
  Phibeta : Outport  Port=2
  wires:
  Valpha/1 -> Subtract/1
  Ialpha/1 -> Gain3/1, Gain/1
  Gain/1 -> Subtract/2
  Subtract/1 -> Add/1  "Y_Alpha"
  Gain1/1 -> Add/2  "NLFcn_Alpha"
  Add/1 -> Gain2/1  "Xdot_Alpha"
  Add1/1 -> Subtract1/1, Delay One Step/1  "X_Alpha"
  Delay One Step/1 -> Add1/2
  Gain2/1 -> Add1/1
  Gain3/1 -> Subtract1/2
  Subtract1/1 -> Phialpha/1, Delay One Step1/1  "Phialpha"
  Product/1 -> Gain1/1
  Delay One Step1/1 -> [Nx_alpha], Product/2
  Delay One Step3/1 -> [Nx_beta], Product1/2
  Product1/1 -> Gain5/1
  Subtract3/1 -> Phibeta/1, Delay One Step3/1  "Phibeta"
  Gain7/1 -> Subtract3/2
  Gain6/1 -> Add3/1
  Delay One Step2/1 -> Add3/2
  Add3/1 -> Delay One Step2/1, Subtract3/1  "X_Beta"
  Add2/1 -> Gain6/1  "Xdot_Beta"
  Gain5/1 -> Add2/2  "NLFcn_Beta"
  Subtract2/1 -> Add2/1  "Y_Beta"
  Gain4/1 -> Subtract2/2
  Ibeta/1 -> Gain4/1, Gain7/1
  Vbeta/1 -> Subtract2/1
  Constant/1 -> Square/1
  [Nx_alpha] -> Square1/1
  [Nx_beta] -> Square2/1
  Square1/1 -> Add4/1
  Square2/1 -> Add4/2
  Square/1 -> Subtract4/1
  Add4/1 -> Subtract4/2  "Psim2"
  Subtract4/1 -> [Nx2]  "Nx2"
  [Nx2] -> Product/1
  [Nx2] -> Product1/1

== system BLAC_MotorCtrl_Math/HFTask/fluxobservor/getSpeedandTheta ==
  Phialpha : Inport
  Phibeta : Inport  Port=2
  Add : Sum
  Add1 : Sum
  Add2 : Sum
  Constant : Constant  Value=2*pi  OutDataTypeStr=single
  Delay One Step : Delay  DelayLength=1
  Delay One Step2 : Delay  DelayLength=1
  Gain : Gain  Gain=1/MC_Motor_Phi
  Gain1 : Gain  Gain=2*sqrt(2)/2*100
  Gain2 : Gain  Gain=100^2*MC_Sim_HFTStep
  Gain3 : Gain  Gain=MC_Param_SpeedtoTheta  OutDataTypeStr=single  RndMeth=Simplest
  Gain4 : Gain  Gain=1/MC_Motor_Phi
  Gain5 : Gain  Gain=30/(pi*MC_Motor_Rotor_Pn)  OutDataTypeStr=single  RndMeth=Simplest
  Mod : Math  Operator=mod
  Product : Product
  Product1 : Product
  Sin : Trigonometry  OutputSignalType=real
  Sin1 : Trigonometry  Operator=cos  OutputSignalType=real
  Subtract : Sum  Inputs=+-
  Speed : Outport
  Theta : Outport  Port=2
  wires:
  [Theta_Last] -> Sin/1, Sin1/1
  Add1/1 -> Gain5/1, Gain3/1  "WeFlux"
  Mod/1 -> Delay One Step2/1, Theta/1  "ThetaFlux"
  Delay One Step2/1 -> [Theta_Last], Add2/2
  Constant/1 -> Mod/2
  Add2/1 -> Mod/1
  Gain3/1 -> Add2/1
  Subtract/1 -> Gain1/1, Gain2/1  "FluxErr"
  Gain1/1 -> Add1/1
  Delay One Step/1 -> Add/2
  Add/1 -> Add1/2, Delay One Step/1
  Gain2/1 -> Add/1
  Product1/1 -> Subtract/2  "FluxSin"
  Product/1 -> Subtract/1  "FluxCos"
  Sin/1 -> Product1/2
  Sin1/1 -> Product/2
  Phibeta/1 -> Gain/1
  Phialpha/1 -> Gain4/1
  Gain/1 -> Product/1
  Gain4/1 -> Product1/1
  Gain5/1 -> Speed/1  "SpeedFlux_RPM"

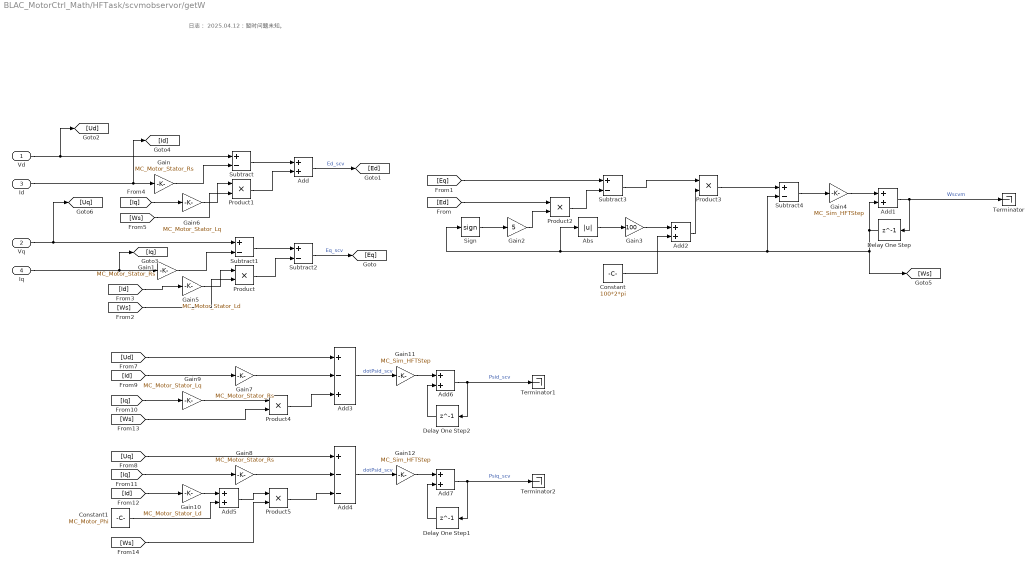
== system BLAC_MotorCtrl_Math/HFTask/scvmobservor/getW ==
  note: 日志：
      | 2025.04.12：暂时问题未知。
  Vd : Inport
  Vq : Inport  Port=2
  Id : Inport  Port=3
  Iq : Inport  Port=4
  Abs : Abs  SaturateOnIntegerOverflow=off
  Add{,1..2,5..7} (6 alike) : Sum
  Add3 : Sum  Inputs=+-+
  Add4 : Sum  Inputs=+--
  Constant : Constant  Value=100*2*pi  OutDataTypeStr=single
  Constant1 : Constant  Value=MC_Motor_Phi  OutDataTypeStr=single
  Delay One Step : Delay  DelayLength=1
  Delay One Step1 : Delay  DelayLength=1
  Delay One Step2 : Delay  DelayLength=1
  Gain{,1,7..8} (4 alike) : Gain  Gain=MC_Motor_Stator_Rs
  Gain10 : Gain  Gain=MC_Motor_Stator_Ld
  Gain11 : Gain  Gain=MC_Sim_HFTStep
  Gain12 : Gain  Gain=MC_Sim_HFTStep
  Gain2 : Gain  Gain=5
  Gain3 : Gain  Gain=100
  Gain4 : Gain  Gain=MC_Sim_HFTStep
  Gain5 : Gain  Gain=MC_Motor_Stator_Ld
  Gain6 : Gain  Gain=MC_Motor_Stator_Lq
  Gain9 : Gain  Gain=MC_Motor_Stator_Lq
  Product{,1..5} (6 alike) : Product
  Sign : Signum
  Subtract{,1..4} (5 alike) : Sum  Inputs=+-
  Terminator : Terminator
  Terminator1 : Terminator
  Terminator2 : Terminator
  wires:
  Id/1 -> [Id], Gain/1
  Gain/1 -> Subtract/2
  Subtract/1 -> Add/1
  Add/1 -> [Ed]  "Ed_scv"
  Gain1/1 -> Subtract1/2
  Iq/1 -> [Iq], Gain1/1
  Vq/1 -> Subtract1/1, [Uq]
  Subtract1/1 -> Subtract2/1
  Product/1 -> Subtract2/2
  Product1/1 -> Add/2
  Subtract2/1 -> [Eq]  "Eq_scv"
  [Ed] -> Product2/1
  Gain2/1 -> Product2/2
  Sign/1 -> Gain2/1
  [Eq] -> Subtract3/1
  Product2/1 -> Subtract3/2
  Subtract3/1 -> Product3/1
  Product3/1 -> Subtract4/1
  Gain4/1 -> Add1/1
  Add1/1 -> Delay One Step/1, Terminator/1  "Wscvm"
  Delay One Step/1 -> [Ws], Subtract4/2, Abs/1, Sign/1, Add1/2
  Subtract4/1 -> Gain4/1
  [Id] -> Gain5/1
  Gain5/1 -> Product/1
  [Ws] -> Product/2
  Gain6/1 -> Product1/1
  [Iq] -> Gain6/1
  [Ws] -> Product1/2
  Abs/1 -> Gain3/1
  Add2/1 -> Product3/2
  Gain3/1 -> Add2/1
  Constant/1 -> Add2/2
  Vd/1 -> Subtract/1, [Ud]
  [Id] -> Gain7/1
  [Iq] -> Gain8/1
  [Ud] -> Add3/1
  Gain7/1 -> Add3/2
  Gain8/1 -> Add4/2
  [Uq] -> Add4/1
  [Ws] -> Product4/2
  Product4/1 -> Add3/3
  Product5/1 -> Add4/3
  [Iq] -> Gain9/1
  Gain9/1 -> Product4/1
  [Id] -> Gain10/1
  Gain10/1 -> Add5/1
  Constant1/1 -> Add5/2
  Add5/1 -> Product5/1
  [Ws] -> Product5/2
  Add3/1 -> Gain11/1  "dotPsid_scv"
  Add4/1 -> Gain12/1  "dotPsid_scv"
  Add7/1 -> Terminator2/1, Delay One Step1/1  "Psiq_scv"
  Delay One Step1/1 -> Add7/2
  Add6/1 -> Terminator1/1, Delay One Step2/1  "Psid_scv"
  Delay One Step2/1 -> Add6/2
  Gain11/1 -> Add6/1
  Gain12/1 -> Add7/1

== system BLAC_MotorCtrl_Math/HFTask/smo/getE ==
  note: 日志：
      | 2025.02.28：滑膜观测器建模无问题，但是反电势观测存在问题，暂时分析为参数问题
  Valpha : Inport
  Vbeta : Inport  Port=2
  Ialpha : Inport  Port=3
  Ibeta : Inport  Port=4
  Add : Sum  Inputs=--+
  Add1 : Sum
  Add2 : Sum  Inputs=+--
  Add3 : Sum
  Delay One Step{,1..3} (4 alike) : Delay  DelayLength=1
  Gain{,4,6,8} (4 alike) : Gain  Gain=MC_Param_SMO_CoffB
  Gain3 : Gain  Gain=MC_Param_SMO_CoffA
  Gain7 : Gain  Gain=MC_Param_SMO_CoffA
  Saturation : Saturate  UpperLimit=100  LowerLimit=-100
  Saturation1 : Saturate  UpperLimit=100  LowerLimit=-100
  Subtract : Sum  Inputs=+-
  Subtract1 : Sum  Inputs=-+
  Ealpha : Outport
  Ebeta : Outport  Port=2
  wires:
  Valpha/1 -> Gain/1
  Add1/1 -> Subtract/1, Delay One Step/1  "Ialpha_SMO"
  Ialpha/1 -> Subtract/2
  Gain/1 -> Add/3
  Gain3/1 -> Add/2
  Gain4/1 -> Add/1
  Delay One Step1/1 -> [Ealpha_SMO]
  [Ialpha_SMO] -> Gain3/1
  [Ealpha_SMO] -> Gain4/1
  Subtract/1 -> Saturation/1
  Saturation/1 -> Ealpha/1, Delay One Step1/1  "Ealpha_SMO"
  Gain6/1 -> Add2/1
  Gain7/1 -> Add2/2
  Gain8/1 -> Add2/3
  Vbeta/1 -> Gain6/1
  Add/1 -> Add1/1  "dotIalpha_SMO"
  Delay One Step/1 -> Add1/2, [Ialpha_SMO]
  Add2/1 -> Add3/2  "dotIbeta_SMO"
  Add3/1 -> Subtract1/2, Delay One Step2/1  "Ibeta_SMO"
  Delay One Step2/1 -> [Ibeta_SMO], Add3/1
  Ibeta/1 -> Subtract1/1
  Subtract1/1 -> Saturation1/1
  Saturation1/1 -> Ebeta/1, Delay One Step3/1  "Ebeta_SMO"
  Delay One Step3/1 -> [Ebeta_SMO]
  [Ibeta_SMO] -> Gain7/1
  [Ebeta_SMO] -> Gain8/1

== system BLAC_MotorCtrl_Math/HFTask/smo/getSpeedandTheta ==
  note: 日志：
      | 2025.03.19：反电势正负号识别错误，改正后可以使用
  Ealpha : Inport
  Ebeta : Inport  Port=2
  Add : Sum
  Add1 : Sum
  Add2 : Sum
  Constant : Constant  Value=2*pi  OutDataTypeStr=single
  Delay One Step : Delay  DelayLength=1
  Delay One Step2 : Delay  DelayLength=1
  Gain : Gain  Gain=-1
  Gain1 : Gain  Gain=2*sqrt(2)/2*100
  Gain2 : Gain  Gain=100^2*MC_Sim_HFTStep
  Gain3 : Gain  Gain=MC_Param_SpeedtoTheta
  Gain5 : Gain  Gain=30/(pi*MC_Motor_Rotor_Pn)  OutDataTypeStr=single  RndMeth=Simplest
  Mod : Math  Operator=mod
  Product : Product
  Product1 : Product
  Sin : Trigonometry  OutputSignalType=real
  Sin1 : Trigonometry  Operator=cos  OutputSignalType=real
  Subtract : Sum  Inputs=+-
  Speed : Outport
  Theta : Outport  Port=2
  wires:
  Sin1/1 -> Product/2
  Sin/1 -> Product1/2
  Gain2/1 -> Add/1
  Add/1 -> Delay One Step/1, Add1/2
  Delay One Step/1 -> Add/2
  Gain1/1 -> Add1/1
  Subtract/1 -> Gain2/1, Gain1/1  "SMOErr"
  Gain3/1 -> Add2/1
  Add2/1 -> Mod/1
  Constant/1 -> Mod/2
  Delay One Step2/1 -> Add2/2, [Theta_Last]
  Mod/1 -> Theta/1, Delay One Step2/1  "ThetaSMO"
  Add1/1 -> Gain5/1, Gain3/1  "SpeedSmo"
  [Theta_Last] -> Sin1/1, Sin/1
  Gain/1 -> Product1/1
  Ebeta/1 -> Gain/1
  Ealpha/1 -> Product/1
  Product/1 -> Subtract/1  "SMOSin"
  Product1/1 -> Subtract/2  "SMOCos"
  Gain5/1 -> Speed/1  "SpeedSMO_RPM"

== system BLAC_MotorCtrl_Math/HFTask/svpwm/getVoltageExchange ==
  Valpha : Inport
  Vbeta : Inport  Port=2
  Vdc : Inport  Port=3
  Add : Sum
  Add1 : Sum
  Divide : Product  Inputs=*/
  Divide1 : Product  Inputs=*/
  Gain : Gain  Gain=-1/2
  Gain1 : Gain  Gain=sqrt(3)/2
  Gain2 : Gain  Gain=-1
  Relational Operator : RelationalOperator  OutDataTypeStr=boolean  RndMeth=Simplest  InputSameDT=off
  Relational Operator1 : RelationalOperator  OutDataTypeStr=boolean  RndMeth=Simplest  InputSameDT=off
  Relational Operator2 : RelationalOperator  Operator=<=  OutDataTypeStr=boolean  RndMeth=Simplest  InputSameDT=off
  Relational Operator3 : RelationalOperator  Operator=<=  OutDataTypeStr=boolean  RndMeth=Simplest  InputSameDT=off
  Signal Copy : SignalConversion  OverrideOpt=off
  Subtract : Sum  Inputs=+-
  Switch{,1..3} (4 alike) : Switch  Criteria=u2 > Threshold  SaturateOnIntegerOverflow=off  InputSameDT=off
  getSectorN : Subsystem  Commented=on
  Va : Outport
  Vb : Outport  Port=2
  Vc : Outport  Port=3
  Vmed : Outport  Port=4
  wires:
  Valpha/1 -> Divide/1
  Vbeta/1 -> Divide1/1
  Vdc/1 -> Divide/2, Divide1/2
  Subtract/1 -> Relational Operator3/2, Switch3/3, Relational Operator1/2, Switch1/3, Vc/1  "Vc"
  Add/1 -> Switch2/3, Relational Operator2/2, Switch/3, Relational Operator/2, Vb/1  "Vb"
  Gain1/1 -> Subtract/2, Add/2
  Gain/1 -> Add/1, Subtract/1
  Divide1/1 -> Gain1/1
  Divide/1 -> Gain/1, Signal Copy/1
  Signal Copy/1 -> Switch2/1, Relational Operator2/1, Switch/1, Relational Operator/1, Va/1  "Va"
  Switch1/1 -> Add1/1  "Vmax"
  Relational Operator1/1 -> Switch1/2
  Switch/1 -> Relational Operator1/1, Switch1/1
  Relational Operator/1 -> Switch/2
  Switch3/1 -> Add1/2  "Vmin"
  Relational Operator3/1 -> Switch3/2
  Switch2/1 -> Switch3/1, Relational Operator3/1
  Relational Operator2/1 -> Switch2/2
  Add1/1 -> Gain2/1
  Gain2/1 -> Vmed/1  "Vmed"

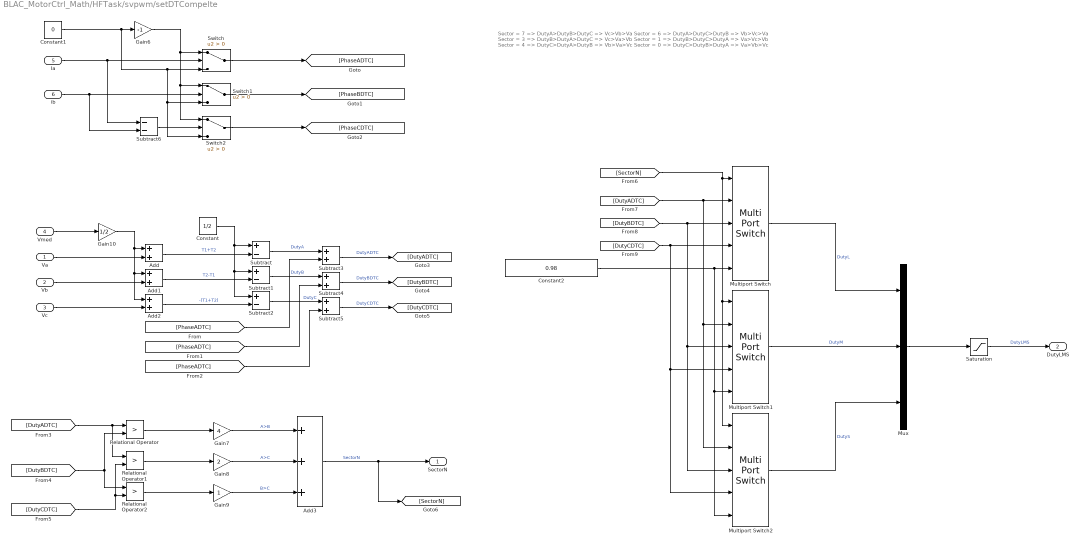
== system BLAC_MotorCtrl_Math/HFTask/svpwm/setDTCompelte ==
  note: Sector = 7 => DutyA>DutyB>DutyC => Vc>Vb>Va
      | Sector = 6 => DutyA>DutyC>DutyB => Vb>Vc>Va
      | Sector = 3 => DutyB>DutyA>DutyC => Vc>Va>Vb
      | Sector = 1 => DutyB>DutyC>DutyA => Va>Vc>Vb
      | Sector = 4 => DutyC>DutyA>DutyB => Vb>Va>Vc
      | Sector = 0 => DutyC>DutyB>DutyA => Va>Vb>Vc
  Va : Inport
  Vb : Inport  Port=2
  Vc : Inport  Port=3
  Vmed : Inport  Port=4
  Ia : Inport  Port=5
  ib : Inport  Port=6
  Add : Sum
  Add1 : Sum
  Add2 : Sum
  Add3 : Sum  Inputs=+++
  Constant : Constant  Value=1/2  OutDataTypeStr=single  SampleTime=MC_Sim_HFTStep
  Constant1 : Constant  Value=0  OutDataTypeStr=single
  Constant2 : Constant  Value=0.98  OutDataTypeStr=single
  Gain10 : Gain  Gain=1/2
  Gain6 : Gain  Gain=-1
  Gain7 : Gain  Gain=4  OutDataTypeStr=single  RndMeth=Simplest
  Gain8 : Gain  Gain=2  OutDataTypeStr=single  RndMeth=Simplest
  Gain9 : Gain  OutDataTypeStr=single  RndMeth=Simplest
  Multiport Switch : MultiPortSwitch  DataPortOrder=Specify indices  DataPortIndices={[6,7],[1,3],[0,4]}  DataPortForDefault=Additional data port  SaturateOnIntegerOverflow=off  InputSameDT=off
  Multiport Switch1 : MultiPortSwitch  DataPortOrder=Specify indices  DataPortIndices={[4,3],[7,0],[6,1]}  DataPortForDefault=Additional data port  SaturateOnIntegerOverflow=off  InputSameDT=off
  Multiport Switch2 : MultiPortSwitch  DataPortOrder=Specify indices  DataPortIndices={[0,1],[4,6],[3,7]}  DataPortForDefault=Additional data port  SaturateOnIntegerOverflow=off  InputSameDT=off
  Mux : Mux  Inputs=3
  Relational Operator : RelationalOperator  Operator=>  OutDataTypeStr=boolean  RndMeth=Simplest  InputSameDT=off
  Relational Operator1 : RelationalOperator  Operator=>  OutDataTypeStr=boolean  RndMeth=Simplest  InputSameDT=off
  Relational Operator2 : RelationalOperator  Operator=>  OutDataTypeStr=boolean  RndMeth=Simplest  InputSameDT=off
  Saturation : Saturate  UpperLimit=0.98  LowerLimit=0.02
      settings: AttributesFormatString=|
      | OutputMax = %<UpperLimit>
      | OutputMin = %<LowerLimit>
  Subtract : Sum  Inputs=+-
  Subtract1 : Sum  Inputs=+-
  Subtract2 : Sum  Inputs=+-
  Subtract3 : Sum
  Subtract4 : Sum
  Subtract5 : Sum
  Subtract6 : Sum  Inputs=--
  Switch : Switch  Criteria=u2 > Threshold  SaturateOnIntegerOverflow=off  InputSameDT=off
  Switch1 : Switch  Criteria=u2 > Threshold  SaturateOnIntegerOverflow=off  InputSameDT=off
  Switch2 : Switch  Criteria=u2 > Threshold  SaturateOnIntegerOverflow=off  InputSameDT=off
  SectorN : Outport
  DutyLMS : Outport  Port=2
  wires:
  Va/1 -> Add/2
  Vmed/1 -> Gain10/1
  Vb/1 -> Add1/2
  Vc/1 -> Add2/2
  Add/1 -> Subtract/2  "T1+T2"
  Add2/1 -> Subtract2/2  "-(T1+T2)"
  Add1/1 -> Subtract1/2  "T2-T1"
  Constant/1 -> Subtract2/1, Subtract1/1, Subtract/1
  Subtract/1 -> Subtract3/1  "DutyA"
  Subtract1/1 -> Subtract4/1  "DutyB"
  Subtract2/1 -> Subtract5/1  "DutyC"
  Ia/1 -> Subtract6/1, Switch/2
  Gain6/1 -> Switch2/1, Switch1/1, Switch/1
  ib/1 -> Subtract6/2, Switch1/2
  Subtract6/1 -> Switch2/2
  Constant1/1 -> Switch2/3, Switch1/3, Switch/3, Gain6/1
  Switch/1 -> [PhaseADTC]
  Switch1/1 -> [PhaseBDTC]
  Switch2/1 -> [PhaseCDTC]
  [PhaseADTC] -> Subtract3/2
  [PhaseADTC] -> Subtract4/2
  [PhaseADTC] -> Subtract5/2
  [DutyBDTC] -> Relational Operator/2, Relational Operator2/1
  [DutyADTC] -> Relational Operator1/1, Relational Operator/1
  [DutyCDTC] -> Relational Operator2/2, Relational Operator1/2
  Relational Operator/1 -> Gain7/1
  Relational Operator1/1 -> Gain8/1
  Relational Operator2/1 -> Gain9/1
  Gain8/1 -> Add3/2  "A>C"
  Gain9/1 -> Add3/3  "B>C"
  Gain7/1 -> Add3/1  "A>B"
  Add3/1 -> [SectorN], SectorN/1  "SectorN"
  Gain10/1 -> Add2/1, Add1/1, Add/1
  Subtract3/1 -> [DutyADTC]  "DutyADTC"
  Subtract4/1 -> [DutyBDTC]  "DutyBDTC"
  Subtract5/1 -> [DutyCDTC]  "DutyCDTC"
  [SectorN] -> Multiport Switch2/1, Multiport Switch1/1, Multiport Switch/1
  Multiport Switch/1 -> Mux/1  "DutyL"
  Constant2/1 -> Multiport Switch2/5, Multiport Switch1/5, Multiport Switch/5
  Multiport Switch1/1 -> Mux/2  "DutyM"
  Multiport Switch2/1 -> Mux/3  "DutyS"
  Mux/1 -> Saturation/1
  Saturation/1 -> DutyLMS/1  "DutyLMS"
  [DutyADTC] -> Multiport Switch2/2, Multiport Switch1/2, Multiport Switch/2
  [DutyCDTC] -> Multiport Switch2/4, Multiport Switch1/4, Multiport Switch/4
  [DutyBDTC] -> Multiport Switch2/3, Multiport Switch1/3, Multiport Switch/3
